simulink library "inp_BCKP"  (R2021b)
settings: Solver=VariableStepAuto  StartTime=0.0  StopTime=10.0  RelTol=1e-3
undefined symbols (not defined in the file): C_TASK_5MS_S, FALSE, KINP_AcoreReadyToSlp_flg_ovrdflg, KINP_AcoreReadyToSlp_flg_ovrdval, KINP_AllowMovThd_OTA_enum_ovrdflg, KINP_AllowMovThd_OTA_enum_ovrdval, KINP_APSAngleTarget_Deg_ovrdflg, KINP_APSAngleTarget_Deg_ovrdval, KINP_APSDecReq_mps2_ovrdflg, KINP_APSDecReq_mps2_ovrdval, KINP_APSDecReqA_flg_ovrdflg, KINP_APSDecReqA_flg_ovrdval, KINP_APSDFLL_cm_ovrdflg, KINP_APSDFLL_cm_ovrdval, KINP_APSDFLR_cm_ovrdflg, KINP_APSDFLR_cm_ovrdval, KINP_APSDRLL_cm_ovrdflg, KINP_APSDRLL_cm_ovrdval, KINP_APSDRLR_cm_ovrdflg, KINP_APSDRLR_cm_ovrdval, KINP_APSExitCondition_enum_ovrdflg, KINP_APSExitCondition_enum_ovrdval, KINP_APSHWVer_enum_ovrdflg, KINP_APSHWVer_enum_ovrdval, KINP_APSProgressPCT_pct_ovrdflg, KINP_APSProgressPCT_pct_ovrdval, KINP_APSPwrReq_enum_ovrdflg, KINP_APSPwrReq_enum_ovrdval, KINP_APSReq_enum_ovrdflg, KINP_APSReq_enum_ovrdval, KINP_APSRQDisplay_enum_ovrdflg, KINP_APSRQDisplay_enum_ovrdval, KINP_APSRqEPASCtrl_flg_ovrdflg, KINP_APSRqEPASCtrl_flg_ovrdval, KINP_APSShiftPosnReq_enum_ovrdval, KINP_APSShiftPosnReq_enum_ovrflg, KINP_APSSpeedCMD_kph_ovrdval, KINP_APSSpeedCMD_kph_ovrflg, KINP_APSStaSystem_enum_ovrdflg, KINP_APSStaSystem_enum_ovrdval, KINP_APSSWVer_enum_ovrdflg, KINP_APSSWVer_enum_ovrdval, KINP_APSVMCReqA_flg_ovrdval, KINP_APSVMCReqA_flg_ovrflg, KINP_APSVRqEPASCtrl_flg_ovrdflg, KINP_APSVRqEPASCtrl_flg_ovrdval, KINP_AuxBattVolmV_mV_ovrdflg, KINP_AuxBattVolmV_mV_ovrdval, KINP_BTConnectSta_enum_ovrdflg, KINP_BTConnectSta_enum_ovrdval, KINP_CAASSta_enum_ovrdflg, KINP_CAASSta_enum_ovrdval, KINP_CAASVMCReqA_flg_ovrdval, KINP_CAASVMCReqA_flg_ovrflg, KINP_CAN1BusOff_flg_ovrdflg, KINP_CAN1BusOff_flg_ovrdval, KINP_CAN2BusOff_flg_ovrdflg, KINP_CAN2BusOff_flg_ovrdval, KINP_CAN3BusOff_flg_ovrdflg, KINP_CAN3BusOff_flg_ovrdval ... (+158)
libraries: FVT_lib x144, hcu_lib x1
(part 6 of 8)

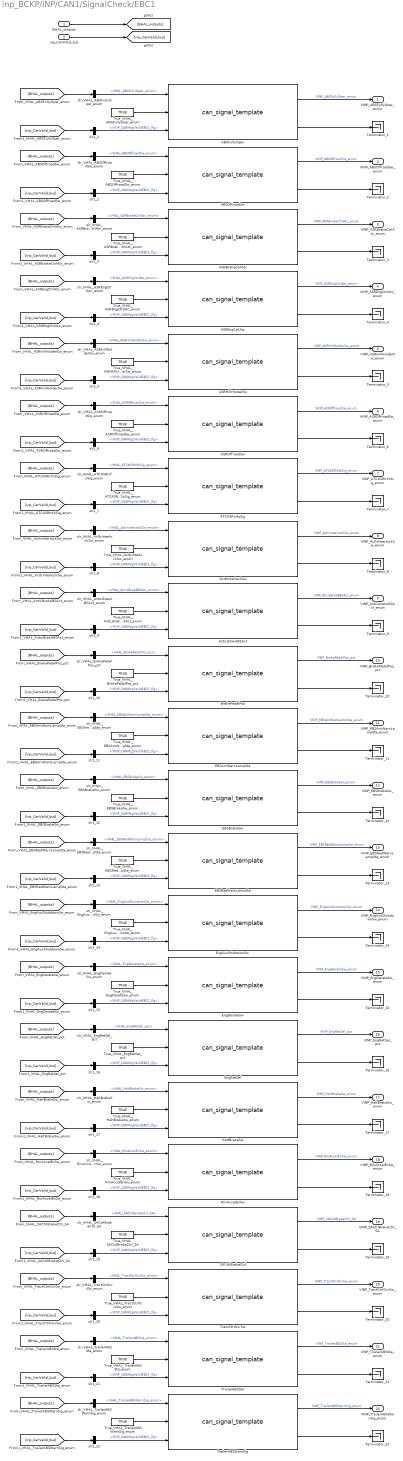
== system inp_BCKP/INP/CAN1/SignalCheck/EBC1 ==
  BHAL_outputs : Inport
  inp_CanValid_bus : Inport  Port=2
  ABSFullyOper : FVT_lib/inp/can_signal_template  SystemSampleTime=-1  VariantActivationTime=update diagram  Latency=0  AutoFrameSizeCalculation=off
      link override defval: Value=KINP_ABSFullyOper_enum_defval
      link override ovrdflg: Value=KINP_ABSFullyOper_enum_ovrdflg
      link override ovrdval: Value=KINP_ABSFullyOper_enum_ovrdval
  ABSOffroadSw : FVT_lib/inp/can_signal_template  SystemSampleTime=-1  VariantActivationTime=update diagram  Latency=0  AutoFrameSizeCalculation=off
      link override defval: Value=KINP_ABSOffroadSw_enum_defval
      link override ovrdflg: Value=KINP_ABSOffroadSw_enum_ovrdflg
      link override ovrdval: Value=KINP_ABSOffroadSw_enum_ovrdval
  ASRBrakeCtrlAtc : FVT_lib/inp/can_signal_template  SystemSampleTime=-1  VariantActivationTime=update diagram  Latency=0  AutoFrameSizeCalculation=off
      link override defval: Value=KINP_ASRBrakeCtrlAtc_enum_defval
      link override ovrdflg: Value=KINP_ASRBrakeCtrlAtc_enum_ovrdflg
      link override ovrdval: Value=KINP_ASRBrakeCtrlAtc_enum_ovrdval
  ASREngCtrlAtc : FVT_lib/inp/can_signal_template  SystemSampleTime=-1  VariantActivationTime=update diagram  Latency=0  AutoFrameSizeCalculation=off
      link override defval: Value=KINP_ASREngCtrlAtc_enum_defval
      link override ovrdflg: Value=KINP_ASREngCtrlAtc_enum_ovrdflg
      link override ovrdval: Value=KINP_ASREngCtrlAtc_enum_ovrdval
  ASRHillHolderSw : FVT_lib/inp/can_signal_template  SystemSampleTime=-1  VariantActivationTime=update diagram  Latency=0  AutoFrameSizeCalculation=off
      link override defval: Value=KINP_ASRHillHolderSw_enum_defval
      link override ovrdflg: Value=KINP_ASRHillHolderSw_enum_ovrdflg
      link override ovrdval: Value=KINP_ASRHillHolderSw_enum_ovrdval
  ASROffroadSw : FVT_lib/inp/can_signal_template  SystemSampleTime=-1  VariantActivationTime=update diagram  Latency=0  AutoFrameSizeCalculation=off
      link override defval: Value=KINP_ASROffroadSw_enum_defval
      link override ovrdflg: Value=KINP_ASROffroadSw_enum_ovrdflg
      link override ovrdval: Value=KINP_ASROffroadSw_enum_ovrdval
  ATCASRInfoSig : FVT_lib/inp/can_signal_template  SystemSampleTime=-1  VariantActivationTime=update diagram  Latency=0  AutoFrameSizeCalculation=off
      link override defval: Value=KINP_ATCASRInfoSig_enum_defval
      link override ovrdflg: Value=KINP_ATCASRInfoSig_enum_ovrdflg
      link override ovrdval: Value=KINP_ATCASRInfoSig_enum_ovrdval
  AcltrInterlockSw : FVT_lib/inp/can_signal_template  SystemSampleTime=-1  VariantActivationTime=update diagram  Latency=0  AutoFrameSizeCalculation=off
      link override defval: Value=KINP_AcltrInterlockSw_enum_defval
      link override ovrdflg: Value=KINP_AcltrInterlockSw_enum_ovrdflg
      link override ovrdval: Value=KINP_AcltrInterlockSw_enum_ovrdval
  AntiLBrakABSAct : FVT_lib/inp/can_signal_template  SystemSampleTime=-1  VariantActivationTime=update diagram  Latency=0  AutoFrameSizeCalculation=off
      link override defval: Value=KINP_AntiLBrakABSAct_enum_defval
      link override ovrdflg: Value=KINP_AntiLBrakABSAct_enum_ovrdflg
      link override ovrdval: Value=KINP_AntiLBrakABSAct_enum_ovrdval
  BrakePedalPos : FVT_lib/inp/can_signal_template  SystemSampleTime=-1  VariantActivationTime=update diagram  Latency=0  AutoFrameSizeCalculation=off
      link override defval: Value=KINP_BrakePedalPos_pct_defval
      link override ovrdflg: Value=KINP_BrakePedalPos_pct_ovrdflg
      link override ovrdval: Value=KINP_BrakePedalPos_pct_ovrdval
  EBSAmWarnLampSta : FVT_lib/inp/can_signal_template  SystemSampleTime=-1  VariantActivationTime=update diagram  Latency=0  AutoFrameSizeCalculation=off
      link override defval: Value=KINP_EBSAmWarnLampSta_enum_defval
      link override ovrdflg: Value=KINP_EBSAmWarnLampSta_enum_ovrdflg
      link override ovrdval: Value=KINP_EBSAmWarnLampSta_enum_ovrdval
  EBSBrakeSw : FVT_lib/inp/can_signal_template  SystemSampleTime=-1  VariantActivationTime=update diagram  Latency=0  AutoFrameSizeCalculation=off
      link override defval: Value=KINP_EBSBrakeSw_enum_defval
      link override ovrdflg: Value=KINP_EBSBrakeSw_enum_ovrdflg
      link override ovrdval: Value=KINP_EBSBrakeSw_enum_ovrdval
  EBSRedWarnLampSta : FVT_lib/inp/can_signal_template  SystemSampleTime=-1  VariantActivationTime=update diagram  Latency=0  AutoFrameSizeCalculation=off
      link override defval: Value=KINP_EBSRedWarnLampSta_enum_defval
      link override ovrdflg: Value=KINP_EBSRedWarnLampSta_enum_ovrdflg
      link override ovrdval: Value=KINP_EBSRedWarnLampSta_enum_ovrdval
  EngAuxShutdownSw : FVT_lib/inp/can_signal_template  SystemSampleTime=-1  VariantActivationTime=update diagram  Latency=0  AutoFrameSizeCalculation=off
      link override defval: Value=KINP_EngAuxShutdownSw_enum_defval
      link override ovrdflg: Value=KINP_EngAuxShutdownSw_enum_ovrdflg
      link override ovrdval: Value=KINP_EngAuxShutdownSw_enum_ovrdval
  EngDerateSw : FVT_lib/inp/can_signal_template  SystemSampleTime=-1  VariantActivationTime=update diagram  Latency=0  AutoFrameSizeCalculation=off
      link override defval: Value=KINP_EngDerateSw_enum_defval
      link override ovrdflg: Value=KINP_EngDerateSw_enum_ovrdflg
      link override ovrdval: Value=KINP_EngDerateSw_enum_ovrdval
  EngRetSel : FVT_lib/inp/can_signal_template  SystemSampleTime=-1  VariantActivationTime=update diagram  Latency=0  AutoFrameSizeCalculation=off
      link override defval: Value=KINP_EngRetSel_pct_defval
      link override ovrdflg: Value=KINP_EngRetSel_pct_ovrdflg
      link override ovrdval: Value=KINP_EngRetSel_pct_ovrdval
  HaltBrakeSw : FVT_lib/inp/can_signal_template  SystemSampleTime=-1  VariantActivationTime=update diagram  Latency=0  AutoFrameSizeCalculation=off
      link override defval: Value=KINP_HaltBrakeSw_enum_defval
      link override ovrdflg: Value=KINP_HaltBrakeSw_enum_ovrdflg
      link override ovrdval: Value=KINP_HaltBrakeSw_enum_ovrdval
  RmAccelEnSw : FVT_lib/inp/can_signal_template  SystemSampleTime=-1  VariantActivationTime=update diagram  Latency=0  AutoFrameSizeCalculation=off
      link override defval: Value=KINP_RmAccelEnSw_enum_defval
      link override ovrdflg: Value=KINP_RmAccelEnSw_enum_ovrdflg
      link override ovrdval: Value=KINP_RmAccelEnSw_enum_ovrdval
  SACtrlBrakeCtrl : FVT_lib/inp/can_signal_template  SystemSampleTime=-1  VariantActivationTime=update diagram  Latency=0  AutoFrameSizeCalculation=off
      link override defval: Value=KINP_SACtrlBrakeCtrl_SA_defval
      link override ovrdflg: Value=KINP_SACtrlBrakeCtrl_SA_ovrdflg
      link override ovrdval: Value=KINP_SACtrlBrakeCtrl_SA_ovrdval
  Terminator_{1..22} (22 alike) : Terminator
  TractCtrlOvrSw : FVT_lib/inp/can_signal_template  SystemSampleTime=-1  VariantActivationTime=update diagram  Latency=0  AutoFrameSizeCalculation=off
      link override defval: Value=KINP_TractCtrlOvrSw_enum_defval
      link override ovrdflg: Value=KINP_TractCtrlOvrSw_enum_ovrdflg
      link override ovrdval: Value=KINP_TractCtrlOvrSw_enum_ovrdval
  TrailerABSSta : FVT_lib/inp/can_signal_template  SystemSampleTime=-1  VariantActivationTime=update diagram  Latency=0  AutoFrameSizeCalculation=off
      link override defval: Value=KINP_TrailerABSSta_enum_defval
      link override ovrdflg: Value=KINP_TrailerABSSta_enum_ovrdflg
      link override ovrdval: Value=KINP_TrailerABSSta_enum_ovrdval
  TrailerABSWarnSig : FVT_lib/inp/can_signal_template  SystemSampleTime=-1  VariantActivationTime=update diagram  Latency=0  AutoFrameSizeCalculation=off
      link override defval: Value=KINP_TrailerABSWarnSig_enum_defval
      link override ovrdflg: Value=KINP_TrailerABSWarnSig_enum_ovrdflg
      link override ovrdval: Value=KINP_TrailerABSWarnSig_enum_ovrdval
  True_VHAL_ABSFullyOper_enum : Constant  Value=TRUE  OutDataTypeStr=boolean
  True_VHAL_ABSOffroadSw_enum : Constant  Value=TRUE  OutDataTypeStr=boolean
  True_VHAL_ASRBrakeCtrlAtc_enum : Constant  Value=TRUE  OutDataTypeStr=boolean
  True_VHAL_ASREngCtrlAtc_enum : Constant  Value=TRUE  OutDataTypeStr=boolean
  True_VHAL_ASRHillHolderSw_enum : Constant  Value=TRUE  OutDataTypeStr=boolean
  True_VHAL_ASROffroadSw_enum : Constant  Value=TRUE  OutDataTypeStr=boolean
  True_VHAL_ATCASRInfoSig_enum : Constant  Value=TRUE  OutDataTypeStr=boolean
  True_VHAL_AcltrInterlockSw_enum : Constant  Value=TRUE  OutDataTypeStr=boolean
  True_VHAL_AntiLBrakABSAct_enum : Constant  Value=TRUE  OutDataTypeStr=boolean
  True_VHAL_BrakePedalPos_pct : Constant  Value=TRUE  OutDataTypeStr=boolean
  True_VHAL_EBSAmWarnLampSta_enum : Constant  Value=TRUE  OutDataTypeStr=boolean
  True_VHAL_EBSBrakeSw_enum : Constant  Value=TRUE  OutDataTypeStr=boolean
  True_VHAL_EBSRedWarnLampSta_enum : Constant  Value=TRUE  OutDataTypeStr=boolean
  True_VHAL_EngAuxShutdownSw_enum : Constant  Value=TRUE  OutDataTypeStr=boolean
  True_VHAL_EngDerateSw_enum : Constant  Value=TRUE  OutDataTypeStr=boolean
  True_VHAL_EngRetSel_pct : Constant  Value=TRUE  OutDataTypeStr=boolean
  True_VHAL_HaltBrakeSw_enum : Constant  Value=TRUE  OutDataTypeStr=boolean
  True_VHAL_RmAccelEnSw_enum : Constant  Value=TRUE  OutDataTypeStr=boolean
  True_VHAL_SACtrlBrakeCtrl_SA : Constant  Value=TRUE  OutDataTypeStr=boolean
  True_VHAL_TractCtrlOvrSw_enum : Constant  Value=TRUE  OutDataTypeStr=boolean
  True_VHAL_TrailerABSSta_enum : Constant  Value=TRUE  OutDataTypeStr=boolean
  True_VHAL_TrailerABSWarnSig_enum : Constant  Value=TRUE  OutDataTypeStr=boolean
  slr1_{1..22} (22 alike) : BusSelector  OutputSignals=VINP_CANMsgValidEBC1_flg
  slr_VHAL_ABSFullyOper_enum : BusSelector  OutputSignals=VHAL_ABSFullyOper_enum
  slr_VHAL_ABSOffroadSw_enum : BusSelector  OutputSignals=VHAL_ABSOffroadSw_enum
  slr_VHAL_ASRBrakeCtrlAtc_enum : BusSelector  OutputSignals=VHAL_ASRBrakeCtrlAtc_enum
  slr_VHAL_ASREngCtrlAtc_enum : BusSelector  OutputSignals=VHAL_ASREngCtrlAtc_enum
  slr_VHAL_ASRHillHolderSw_enum : BusSelector  OutputSignals=VHAL_ASRHillHolderSw_enum
  slr_VHAL_ASROffroadSw_enum : BusSelector  OutputSignals=VHAL_ASROffroadSw_enum
  slr_VHAL_ATCASRInfoSig_enum : BusSelector  OutputSignals=VHAL_ATCASRInfoSig_enum
  slr_VHAL_AcltrInterlockSw_enum : BusSelector  OutputSignals=VHAL_AcltrInterlockSw_enum
  slr_VHAL_AntiLBrakABSAct_enum : BusSelector  OutputSignals=VHAL_AntiLBrakABSAct_enum
  slr_VHAL_BrakePedalPos_pct : BusSelector  OutputSignals=VHAL_BrakePedalPos_pct
  slr_VHAL_EBSAmWarnLampSta_enum : BusSelector  OutputSignals=VHAL_EBSAmWarnLampSta_enum
  slr_VHAL_EBSBrakeSw_enum : BusSelector  OutputSignals=VHAL_EBSBrakeSw_enum
  slr_VHAL_EBSRedWarnLampSta_enum : BusSelector  OutputSignals=VHAL_EBSRedWarnLampSta_enum
  slr_VHAL_EngAuxShutdownSw_enum : BusSelector  OutputSignals=VHAL_EngAuxShutdownSw_enum
  slr_VHAL_EngDerateSw_enum : BusSelector  OutputSignals=VHAL_EngDerateSw_enum
  slr_VHAL_EngRetSel_pct : BusSelector  OutputSignals=VHAL_EngRetSel_pct
  slr_VHAL_HaltBrakeSw_enum : BusSelector  OutputSignals=VHAL_HaltBrakeSw_enum
  slr_VHAL_RmAccelEnSw_enum : BusSelector  OutputSignals=VHAL_RmAccelEnSw_enum
  slr_VHAL_SACtrlBrakeCtrl_SA : BusSelector  OutputSignals=VHAL_SACtrlBrakeCtrl_SA
  slr_VHAL_TractCtrlOvrSw_enum : BusSelector  OutputSignals=VHAL_TractCtrlOvrSw_enum
  slr_VHAL_TrailerABSSta_enum : BusSelector  OutputSignals=VHAL_TrailerABSSta_enum
  slr_VHAL_TrailerABSWarnSig_enum : BusSelector  OutputSignals=VHAL_TrailerABSWarnSig_enum
  VINP_ABSFullyOper_enum : Outport
  VINP_ABSOffroadSw_enum : Outport  Port=2
  VINP_ASRBrakeCtrlAtc_enum : Outport  Port=3
  VINP_ASREngCtrlAtc_enum : Outport  Port=4
  VINP_ASRHillHolderSw_enum : Outport  Port=5
  VINP_ASROffroadSw_enum : Outport  Port=6
  VINP_ATCASRInfoSig_enum : Outport  Port=7
  VINP_AcltrInterlockSw_enum : Outport  Port=8
  VINP_AntiLBrakABSAct_enum : Outport  Port=9
  VINP_BrakePedalPos_pct : Outport  Port=10
  VINP_EBSAmWarnLampSta_enum : Outport  Port=11
  VINP_EBSBrakeSw_enum : Outport  Port=12
  VINP_EBSRedWarnLampSta_enum : Outport  Port=13
  VINP_EngAuxShutdownSw_enum : Outport  Port=14
  VINP_EngDerateSw_enum : Outport  Port=15
  VINP_EngRetSel_pct : Outport  Port=16
  VINP_HaltBrakeSw_enum : Outport  Port=17
  VINP_RmAccelEnSw_enum : Outport  Port=18
  VINP_SACtrlBrakeCtrl_SA : Outport  Port=19
  VINP_TractCtrlOvrSw_enum : Outport  Port=20
  VINP_TrailerABSSta_enum : Outport  Port=21
  VINP_TrailerABSWarnSig_enum : Outport  Port=22
  wires:
  BHAL_outputs/1 -> [BHAL_outputs]
  inp_CanValid_bus/1 -> [inp_CanValid_bus]
  [BHAL_outputs] -> slr_VHAL_ABSFullyOper_enum/1
  slr_VHAL_ABSFullyOper_enum/1 -> ABSFullyOper/1  "<VHAL_ABSFullyOper_enum>"
  True_VHAL_ABSFullyOper_enum/1 -> ABSFullyOper/2
  [inp_CanValid_bus] -> slr1_1/1
  slr1_1/1 -> ABSFullyOper/3  "<VINP_CANMsgValidEBC1_flg>"
  ABSFullyOper/1 -> VINP_ABSFullyOper_enum/1  "VINP_ABSFullyOper_enum"
  ABSFullyOper/2 -> Terminator_1/1
  [BHAL_outputs] -> slr_VHAL_ABSOffroadSw_enum/1
  slr_VHAL_ABSOffroadSw_enum/1 -> ABSOffroadSw/1  "<VHAL_ABSOffroadSw_enum>"
  True_VHAL_ABSOffroadSw_enum/1 -> ABSOffroadSw/2
  [inp_CanValid_bus] -> slr1_2/1
  slr1_2/1 -> ABSOffroadSw/3  "<VINP_CANMsgValidEBC1_flg>"
  ABSOffroadSw/1 -> VINP_ABSOffroadSw_enum/1  "VINP_ABSOffroadSw_enum"
  ABSOffroadSw/2 -> Terminator_2/1
  [BHAL_outputs] -> slr_VHAL_ASRBrakeCtrlAtc_enum/1
  slr_VHAL_ASRBrakeCtrlAtc_enum/1 -> ASRBrakeCtrlAtc/1  "<VHAL_ASRBrakeCtrlAtc_enum>"
  True_VHAL_ASRBrakeCtrlAtc_enum/1 -> ASRBrakeCtrlAtc/2
  [inp_CanValid_bus] -> slr1_3/1
  slr1_3/1 -> ASRBrakeCtrlAtc/3  "<VINP_CANMsgValidEBC1_flg>"
  ASRBrakeCtrlAtc/1 -> VINP_ASRBrakeCtrlAtc_enum/1  "VINP_ASRBrakeCtrlAtc_enum"
  ASRBrakeCtrlAtc/2 -> Terminator_3/1
  [BHAL_outputs] -> slr_VHAL_ASREngCtrlAtc_enum/1
  slr_VHAL_ASREngCtrlAtc_enum/1 -> ASREngCtrlAtc/1  "<VHAL_ASREngCtrlAtc_enum>"
  True_VHAL_ASREngCtrlAtc_enum/1 -> ASREngCtrlAtc/2
  [inp_CanValid_bus] -> slr1_4/1
  slr1_4/1 -> ASREngCtrlAtc/3  "<VINP_CANMsgValidEBC1_flg>"
  ASREngCtrlAtc/1 -> VINP_ASREngCtrlAtc_enum/1  "VINP_ASREngCtrlAtc_enum"
  ASREngCtrlAtc/2 -> Terminator_4/1
  [BHAL_outputs] -> slr_VHAL_ASRHillHolderSw_enum/1
  slr_VHAL_ASRHillHolderSw_enum/1 -> ASRHillHolderSw/1  "<VHAL_ASRHillHolderSw_enum>"
  True_VHAL_ASRHillHolderSw_enum/1 -> ASRHillHolderSw/2
  [inp_CanValid_bus] -> slr1_5/1
  slr1_5/1 -> ASRHillHolderSw/3  "<VINP_CANMsgValidEBC1_flg>"
  ASRHillHolderSw/1 -> VINP_ASRHillHolderSw_enum/1  "VINP_ASRHillHolderSw_enum"
  ASRHillHolderSw/2 -> Terminator_5/1
  [BHAL_outputs] -> slr_VHAL_ASROffroadSw_enum/1
  slr_VHAL_ASROffroadSw_enum/1 -> ASROffroadSw/1  "<VHAL_ASROffroadSw_enum>"
  True_VHAL_ASROffroadSw_enum/1 -> ASROffroadSw/2
  [inp_CanValid_bus] -> slr1_6/1
  slr1_6/1 -> ASROffroadSw/3  "<VINP_CANMsgValidEBC1_flg>"
  ASROffroadSw/1 -> VINP_ASROffroadSw_enum/1  "VINP_ASROffroadSw_enum"
  ASROffroadSw/2 -> Terminator_6/1
  [BHAL_outputs] -> slr_VHAL_ATCASRInfoSig_enum/1
  slr_VHAL_ATCASRInfoSig_enum/1 -> ATCASRInfoSig/1  "<VHAL_ATCASRInfoSig_enum>"
  True_VHAL_ATCASRInfoSig_enum/1 -> ATCASRInfoSig/2
  [inp_CanValid_bus] -> slr1_7/1
  slr1_7/1 -> ATCASRInfoSig/3  "<VINP_CANMsgValidEBC1_flg>"
  ATCASRInfoSig/1 -> VINP_ATCASRInfoSig_enum/1  "VINP_ATCASRInfoSig_enum"
  ATCASRInfoSig/2 -> Terminator_7/1
  [BHAL_outputs] -> slr_VHAL_AcltrInterlockSw_enum/1
  slr_VHAL_AcltrInterlockSw_enum/1 -> AcltrInterlockSw/1  "<VHAL_AcltrInterlockSw_enum>"
  True_VHAL_AcltrInterlockSw_enum/1 -> AcltrInterlockSw/2
  [inp_CanValid_bus] -> slr1_8/1
  slr1_8/1 -> AcltrInterlockSw/3  "<VINP_CANMsgValidEBC1_flg>"
  AcltrInterlockSw/1 -> VINP_AcltrInterlockSw_enum/1  "VINP_AcltrInterlockSw_enum"
  AcltrInterlockSw/2 -> Terminator_8/1
  [BHAL_outputs] -> slr_VHAL_AntiLBrakABSAct_enum/1
  slr_VHAL_AntiLBrakABSAct_enum/1 -> AntiLBrakABSAct/1  "<VHAL_AntiLBrakABSAct_enum>"
  True_VHAL_AntiLBrakABSAct_enum/1 -> AntiLBrakABSAct/2
  [inp_CanValid_bus] -> slr1_9/1
  slr1_9/1 -> AntiLBrakABSAct/3  "<VINP_CANMsgValidEBC1_flg>"
  AntiLBrakABSAct/1 -> VINP_AntiLBrakABSAct_enum/1  "VINP_AntiLBrakABSAct_enum"
  AntiLBrakABSAct/2 -> Terminator_9/1
  [BHAL_outputs] -> slr_VHAL_BrakePedalPos_pct/1
  slr_VHAL_BrakePedalPos_pct/1 -> BrakePedalPos/1  "<VHAL_BrakePedalPos_pct>"
  True_VHAL_BrakePedalPos_pct/1 -> BrakePedalPos/2
  [inp_CanValid_bus] -> slr1_10/1
  slr1_10/1 -> BrakePedalPos/3  "<VINP_CANMsgValidEBC1_flg>"
  BrakePedalPos/1 -> VINP_BrakePedalPos_pct/1  "VINP_BrakePedalPos_pct"
  BrakePedalPos/2 -> Terminator_10/1
  [BHAL_outputs] -> slr_VHAL_EBSAmWarnLampSta_enum/1
  slr_VHAL_EBSAmWarnLampSta_enum/1 -> EBSAmWarnLampSta/1  "<VHAL_EBSAmWarnLampSta_enum>"
  True_VHAL_EBSAmWarnLampSta_enum/1 -> EBSAmWarnLampSta/2
  [inp_CanValid_bus] -> slr1_11/1
  slr1_11/1 -> EBSAmWarnLampSta/3  "<VINP_CANMsgValidEBC1_flg>"
  EBSAmWarnLampSta/1 -> VINP_EBSAmWarnLampSta_enum/1  "VINP_EBSAmWarnLampSta_enum"
  EBSAmWarnLampSta/2 -> Terminator_11/1
  [BHAL_outputs] -> slr_VHAL_EBSBrakeSw_enum/1
  slr_VHAL_EBSBrakeSw_enum/1 -> EBSBrakeSw/1  "<VHAL_EBSBrakeSw_enum>"
  True_VHAL_EBSBrakeSw_enum/1 -> EBSBrakeSw/2
  [inp_CanValid_bus] -> slr1_12/1
  slr1_12/1 -> EBSBrakeSw/3  "<VINP_CANMsgValidEBC1_flg>"
  EBSBrakeSw/1 -> VINP_EBSBrakeSw_enum/1  "VINP_EBSBrakeSw_enum"
  EBSBrakeSw/2 -> Terminator_12/1
  [BHAL_outputs] -> slr_VHAL_EBSRedWarnLampSta_enum/1
  slr_VHAL_EBSRedWarnLampSta_enum/1 -> EBSRedWarnLampSta/1  "<VHAL_EBSRedWarnLampSta_enum>"
  True_VHAL_EBSRedWarnLampSta_enum/1 -> EBSRedWarnLampSta/2
  [inp_CanValid_bus] -> slr1_13/1
  slr1_13/1 -> EBSRedWarnLampSta/3  "<VINP_CANMsgValidEBC1_flg>"
  EBSRedWarnLampSta/1 -> VINP_EBSRedWarnLampSta_enum/1  "VINP_EBSRedWarnLampSta_enum"
  EBSRedWarnLampSta/2 -> Terminator_13/1
  [BHAL_outputs] -> slr_VHAL_EngAuxShutdownSw_enum/1
  slr_VHAL_EngAuxShutdownSw_enum/1 -> EngAuxShutdownSw/1  "<VHAL_EngAuxShutdownSw_enum>"
  True_VHAL_EngAuxShutdownSw_enum/1 -> EngAuxShutdownSw/2
  [inp_CanValid_bus] -> slr1_14/1
  slr1_14/1 -> EngAuxShutdownSw/3  "<VINP_CANMsgValidEBC1_flg>"
  EngAuxShutdownSw/1 -> VINP_EngAuxShutdownSw_enum/1  "VINP_EngAuxShutdownSw_enum"
  EngAuxShutdownSw/2 -> Terminator_14/1
  [BHAL_outputs] -> slr_VHAL_EngDerateSw_enum/1
  slr_VHAL_EngDerateSw_enum/1 -> EngDerateSw/1  "<VHAL_EngDerateSw_enum>"
  True_VHAL_EngDerateSw_enum/1 -> EngDerateSw/2
  [inp_CanValid_bus] -> slr1_15/1
  slr1_15/1 -> EngDerateSw/3  "<VINP_CANMsgValidEBC1_flg>"
  EngDerateSw/1 -> VINP_EngDerateSw_enum/1  "VINP_EngDerateSw_enum"
  EngDerateSw/2 -> Terminator_15/1
  [BHAL_outputs] -> slr_VHAL_EngRetSel_pct/1
  slr_VHAL_EngRetSel_pct/1 -> EngRetSel/1  "<VHAL_EngRetSel_pct>"
  True_VHAL_EngRetSel_pct/1 -> EngRetSel/2
  [inp_CanValid_bus] -> slr1_16/1
  slr1_16/1 -> EngRetSel/3  "<VINP_CANMsgValidEBC1_flg>"
  EngRetSel/1 -> VINP_EngRetSel_pct/1  "VINP_EngRetSel_pct"
  EngRetSel/2 -> Terminator_16/1
  [BHAL_outputs] -> slr_VHAL_HaltBrakeSw_enum/1
  slr_VHAL_HaltBrakeSw_enum/1 -> HaltBrakeSw/1  "<VHAL_HaltBrakeSw_enum>"
  True_VHAL_HaltBrakeSw_enum/1 -> HaltBrakeSw/2
  [inp_CanValid_bus] -> slr1_17/1
  slr1_17/1 -> HaltBrakeSw/3  "<VINP_CANMsgValidEBC1_flg>"
  HaltBrakeSw/1 -> VINP_HaltBrakeSw_enum/1  "VINP_HaltBrakeSw_enum"
  HaltBrakeSw/2 -> Terminator_17/1
  [BHAL_outputs] -> slr_VHAL_RmAccelEnSw_enum/1
  slr_VHAL_RmAccelEnSw_enum/1 -> RmAccelEnSw/1  "<VHAL_RmAccelEnSw_enum>"
  True_VHAL_RmAccelEnSw_enum/1 -> RmAccelEnSw/2
  [inp_CanValid_bus] -> slr1_18/1
  slr1_18/1 -> RmAccelEnSw/3  "<VINP_CANMsgValidEBC1_flg>"
  RmAccelEnSw/1 -> VINP_RmAccelEnSw_enum/1  "VINP_RmAccelEnSw_enum"
  RmAccelEnSw/2 -> Terminator_18/1
  [BHAL_outputs] -> slr_VHAL_SACtrlBrakeCtrl_SA/1
  slr_VHAL_SACtrlBrakeCtrl_SA/1 -> SACtrlBrakeCtrl/1  "<VHAL_SACtrlBrakeCtrl_SA>"
  True_VHAL_SACtrlBrakeCtrl_SA/1 -> SACtrlBrakeCtrl/2
  [inp_CanValid_bus] -> slr1_19/1
  slr1_19/1 -> SACtrlBrakeCtrl/3  "<VINP_CANMsgValidEBC1_flg>"
  SACtrlBrakeCtrl/1 -> VINP_SACtrlBrakeCtrl_SA/1  "VINP_SACtrlBrakeCtrl_SA"
  SACtrlBrakeCtrl/2 -> Terminator_19/1
  [BHAL_outputs] -> slr_VHAL_TractCtrlOvrSw_enum/1
  slr_VHAL_TractCtrlOvrSw_enum/1 -> TractCtrlOvrSw/1  "<VHAL_TractCtrlOvrSw_enum>"
  True_VHAL_TractCtrlOvrSw_enum/1 -> TractCtrlOvrSw/2
  [inp_CanValid_bus] -> slr1_20/1
  slr1_20/1 -> TractCtrlOvrSw/3  "<VINP_CANMsgValidEBC1_flg>"
  TractCtrlOvrSw/1 -> VINP_TractCtrlOvrSw_enum/1  "VINP_TractCtrlOvrSw_enum"
  TractCtrlOvrSw/2 -> Terminator_20/1
  [BHAL_outputs] -> slr_VHAL_TrailerABSSta_enum/1
  slr_VHAL_TrailerABSSta_enum/1 -> TrailerABSSta/1  "<VHAL_TrailerABSSta_enum>"
  True_VHAL_TrailerABSSta_enum/1 -> TrailerABSSta/2
  [inp_CanValid_bus] -> slr1_21/1
  slr1_21/1 -> TrailerABSSta/3  "<VINP_CANMsgValidEBC1_flg>"
  TrailerABSSta/1 -> VINP_TrailerABSSta_enum/1  "VINP_TrailerABSSta_enum"
  TrailerABSSta/2 -> Terminator_21/1
  [BHAL_outputs] -> slr_VHAL_TrailerABSWarnSig_enum/1
  slr_VHAL_TrailerABSWarnSig_enum/1 -> TrailerABSWarnSig/1  "<VHAL_TrailerABSWarnSig_enum>"
  True_VHAL_TrailerABSWarnSig_enum/1 -> TrailerABSWarnSig/2
  [inp_CanValid_bus] -> slr1_22/1
  slr1_22/1 -> TrailerABSWarnSig/3  "<VINP_CANMsgValidEBC1_flg>"
  TrailerABSWarnSig/1 -> VINP_TrailerABSWarnSig_enum/1  "VINP_TrailerABSWarnSig_enum"
  TrailerABSWarnSig/2 -> Terminator_22/1

== system inp_BCKP/INP/CAN1/SignalCheck/EBC2 ==
  BHAL_outputs : Inport
  inp_CanValid_bus : Inport  Port=2
  FASpeed : FVT_lib/inp/can_signal_template  SystemSampleTime=-1  VariantActivationTime=update diagram  Latency=0  AutoFrameSizeCalculation=off
      link override defval: Value=KINP_FASpeed_kph_defval
      link override ovrdflg: Value=KINP_FASpeed_kph_ovrdflg
      link override ovrdval: Value=KINP_FASpeed_kph_ovrdval
  RelaSpdFALWheel : FVT_lib/inp/can_signal_template  SystemSampleTime=-1  VariantActivationTime=update diagram  Latency=0  AutoFrameSizeCalculation=off
      link override defval: Value=KINP_RelaSpdFALWheel_kph_defval
      link override ovrdflg: Value=KINP_RelaSpdFALWheel_kph_ovrdflg
      link override ovrdval: Value=KINP_RelaSpdFALWheel_kph_ovrdval
  RelaSpdFARWheel : FVT_lib/inp/can_signal_template  SystemSampleTime=-1  VariantActivationTime=update diagram  Latency=0  AutoFrameSizeCalculation=off
      link override defval: Value=KINP_RelaSpdFARWheel_kph_defval
      link override ovrdflg: Value=KINP_RelaSpdFARWheel_kph_ovrdflg
      link override ovrdval: Value=KINP_RelaSpdFARWheel_kph_ovrdval
  Terminator_1 : Terminator
  Terminator_2 : Terminator
  Terminator_3 : Terminator
  True_VHAL_FASpeed_kph : Constant  Value=TRUE  OutDataTypeStr=boolean
  True_VHAL_RelaSpdFALWheel_kph : Constant  Value=TRUE  OutDataTypeStr=boolean
  True_VHAL_RelaSpdFARWheel_kph : Constant  Value=TRUE  OutDataTypeStr=boolean
  slr1_1 : BusSelector  OutputSignals=VINP_CANMsgValidEBC2_flg
  slr1_2 : BusSelector  OutputSignals=VINP_CANMsgValidEBC2_flg
  slr1_3 : BusSelector  OutputSignals=VINP_CANMsgValidEBC2_flg
  slr_VHAL_FASpeed_kph : BusSelector  OutputSignals=VHAL_FASpeed_kph
  slr_VHAL_RelaSpdFALWheel_kph : BusSelector  OutputSignals=VHAL_RelaSpdFALWheel_kph
  slr_VHAL_RelaSpdFARWheel_kph : BusSelector  OutputSignals=VHAL_RelaSpdFARWheel_kph
  VINP_FASpeed_kph : Outport
  VINP_RelaSpdFALWheel_kph : Outport  Port=2
  VINP_RelaSpdFARWheel_kph : Outport  Port=3
  wires:
  BHAL_outputs/1 -> [BHAL_outputs]
  inp_CanValid_bus/1 -> [inp_CanValid_bus]
  [BHAL_outputs] -> slr_VHAL_FASpeed_kph/1
  slr_VHAL_FASpeed_kph/1 -> FASpeed/1  "<VHAL_FASpeed_kph>"
  True_VHAL_FASpeed_kph/1 -> FASpeed/2
  [inp_CanValid_bus] -> slr1_1/1
  slr1_1/1 -> FASpeed/3  "<VINP_CANMsgValidEBC2_flg>"
  FASpeed/1 -> VINP_FASpeed_kph/1  "VINP_FASpeed_kph"
  FASpeed/2 -> Terminator_1/1
  [BHAL_outputs] -> slr_VHAL_RelaSpdFALWheel_kph/1
  slr_VHAL_RelaSpdFALWheel_kph/1 -> RelaSpdFALWheel/1  "<VHAL_RelaSpdFALWheel_kph>"
  True_VHAL_RelaSpdFALWheel_kph/1 -> RelaSpdFALWheel/2
  [inp_CanValid_bus] -> slr1_2/1
  slr1_2/1 -> RelaSpdFALWheel/3  "<VINP_CANMsgValidEBC2_flg>"
  RelaSpdFALWheel/1 -> VINP_RelaSpdFALWheel_kph/1  "VINP_RelaSpdFALWheel_kph"
  RelaSpdFALWheel/2 -> Terminator_2/1
  [BHAL_outputs] -> slr_VHAL_RelaSpdFARWheel_kph/1
  slr_VHAL_RelaSpdFARWheel_kph/1 -> RelaSpdFARWheel/1  "<VHAL_RelaSpdFARWheel_kph>"
  True_VHAL_RelaSpdFARWheel_kph/1 -> RelaSpdFARWheel/2
  [inp_CanValid_bus] -> slr1_3/1
  slr1_3/1 -> RelaSpdFARWheel/3  "<VINP_CANMsgValidEBC2_flg>"
  RelaSpdFARWheel/1 -> VINP_RelaSpdFARWheel_kph/1  "VINP_RelaSpdFARWheel_kph"
  RelaSpdFARWheel/2 -> Terminator_3/1

== system inp_BCKP/INP/CAN1/SignalCheck/EBC5 ==
  BHAL_outputs : Inport
  inp_CanValid_bus : Inport  Port=2
  BrkTempeWarn : FVT_lib/inp/can_signal_template  SystemSampleTime=-1  VariantActivationTime=update diagram  Latency=0  AutoFrameSizeCalculation=off
      link override defval: Value=KINP_BrkTempeWarn_enum_defval
      link override ovrdflg: Value=KINP_BrkTempeWarn_enum_ovrdflg
      link override ovrdval: Value=KINP_BrkTempeWarn_enum_ovrdval
  FndBrkUse : FVT_lib/inp/can_signal_template  SystemSampleTime=-1  VariantActivationTime=update diagram  Latency=0  AutoFrameSizeCalculation=off
      link override defval: Value=KINP_FndBrkUse_enum_defval
      link override ovrdflg: Value=KINP_FndBrkUse_enum_ovrdflg
      link override ovrdval: Value=KINP_FndBrkUse_enum_ovrdval
  HaltBrkMode : FVT_lib/inp/can_signal_template  SystemSampleTime=-1  VariantActivationTime=update diagram  Latency=0  AutoFrameSizeCalculation=off
      link override defval: Value=KINP_HaltBrkMode_enum_defval
      link override ovrdflg: Value=KINP_HaltBrkMode_enum_ovrdflg
      link override ovrdval: Value=KINP_HaltBrkMode_enum_ovrdval
  HillHolderMode : FVT_lib/inp/can_signal_template  SystemSampleTime=-1  VariantActivationTime=update diagram  Latency=0  AutoFrameSizeCalculation=off
      link override defval: Value=KINP_HillHolderMode_enum_defval
      link override ovrdflg: Value=KINP_HillHolderMode_enum_ovrdflg
      link override ovrdval: Value=KINP_HillHolderMode_enum_ovrdval
  ParkBrkActuFAct : FVT_lib/inp/can_signal_template  SystemSampleTime=-1  VariantActivationTime=update diagram  Latency=0  AutoFrameSizeCalculation=off
      link override defval: Value=KINP_ParkBrkActuFAct_enum_defval
      link override ovrdflg: Value=KINP_ParkBrkActuFAct_enum_ovrdflg
      link override ovrdval: Value=KINP_ParkBrkActuFAct_enum_ovrdval
  Terminator_{1..8} (8 alike) : Terminator
  True_VHAL_BrkTempeWarn_enum : Constant  Value=TRUE  OutDataTypeStr=boolean
  True_VHAL_FndBrkUse_enum : Constant  Value=TRUE  OutDataTypeStr=boolean
  True_VHAL_HaltBrkMode_enum : Constant  Value=TRUE  OutDataTypeStr=boolean
  True_VHAL_HillHolderMode_enum : Constant  Value=TRUE  OutDataTypeStr=boolean
  True_VHAL_ParkBrkActuFAct_enum : Constant  Value=TRUE  OutDataTypeStr=boolean
  True_VHAL_XBRAcltnLimit_mps2 : Constant  Value=TRUE  OutDataTypeStr=boolean
  True_VHAL_XBRActtrlMode_enum : Constant  Value=TRUE  OutDataTypeStr=boolean
  True_VHAL_XBRSysSta_enum : Constant  Value=TRUE  OutDataTypeStr=boolean
  XBRAcltnLimit : FVT_lib/inp/can_signal_template  SystemSampleTime=-1  VariantActivationTime=update diagram  Latency=0  AutoFrameSizeCalculation=off
      link override defval: Value=KINP_XBRAcltnLimit_mps2_defval
      link override ovrdflg: Value=KINP_XBRAcltnLimit_mps2_ovrdflg
      link override ovrdval: Value=KINP_XBRAcltnLimit_mps2_ovrdval
  XBRActtrlMode : FVT_lib/inp/can_signal_template  SystemSampleTime=-1  VariantActivationTime=update diagram  Latency=0  AutoFrameSizeCalculation=off
      link override defval: Value=KINP_XBRActtrlMode_enum_defval
      link override ovrdflg: Value=KINP_XBRActtrlMode_enum_ovrdflg
      link override ovrdval: Value=KINP_XBRActtrlMode_enum_ovrdval
  XBRSysSta : FVT_lib/inp/can_signal_template  SystemSampleTime=-1  VariantActivationTime=update diagram  Latency=0  AutoFrameSizeCalculation=off
      link override defval: Value=KINP_XBRSysSta_enum_defval
      link override ovrdflg: Value=KINP_XBRSysSta_enum_ovrdflg
      link override ovrdval: Value=KINP_XBRSysSta_enum_ovrdval
  slr1_{1..8} (8 alike) : BusSelector  OutputSignals=VINP_CANMsgValidEBC5_flg
  slr_VHAL_BrkTempeWarn_enum : BusSelector  OutputSignals=VHAL_BrkTempeWarn_enum
  slr_VHAL_FndBrkUse_enum : BusSelector  OutputSignals=VHAL_FndBrkUse_enum
  slr_VHAL_HaltBrkMode_enum : BusSelector  OutputSignals=VHAL_HaltBrkMode_enum
  slr_VHAL_HillHolderMode_enum : BusSelector  OutputSignals=VHAL_HillHolderMode_enum
  slr_VHAL_ParkBrkActuFAct_enum : BusSelector  OutputSignals=VHAL_ParkBrkActuFAct_enum
  slr_VHAL_XBRAcltnLimit_mps2 : BusSelector  OutputSignals=VHAL_XBRAcltnLimit_mps2
  slr_VHAL_XBRActtrlMode_enum : BusSelector  OutputSignals=VHAL_XBRActtrlMode_enum
  slr_VHAL_XBRSysSta_enum : BusSelector  OutputSignals=VHAL_XBRSysSta_enum
  VINP_BrkTempeWarn_enum : Outport
  VINP_FndBrkUse_enum : Outport  Port=2
  VINP_HaltBrkMode_enum : Outport  Port=3
  VINP_HillHolderMode_enum : Outport  Port=4
  VINP_ParkBrkActuFAct_enum : Outport  Port=5
  VINP_XBRAcltnLimit_mps2 : Outport  Port=6
  VINP_XBRActtrlMode_enum : Outport  Port=7
  VINP_XBRSysSta_enum : Outport  Port=8
  wires:
  BHAL_outputs/1 -> [BHAL_outputs]
  inp_CanValid_bus/1 -> [inp_CanValid_bus]
  [BHAL_outputs] -> slr_VHAL_BrkTempeWarn_enum/1
  slr_VHAL_BrkTempeWarn_enum/1 -> BrkTempeWarn/1  "<VHAL_BrkTempeWarn_enum>"
  True_VHAL_BrkTempeWarn_enum/1 -> BrkTempeWarn/2
  [inp_CanValid_bus] -> slr1_1/1
  slr1_1/1 -> BrkTempeWarn/3  "<VINP_CANMsgValidEBC5_flg>"
  BrkTempeWarn/1 -> VINP_BrkTempeWarn_enum/1  "VINP_BrkTempeWarn_enum"
  BrkTempeWarn/2 -> Terminator_1/1
  [BHAL_outputs] -> slr_VHAL_FndBrkUse_enum/1
  slr_VHAL_FndBrkUse_enum/1 -> FndBrkUse/1  "<VHAL_FndBrkUse_enum>"
  True_VHAL_FndBrkUse_enum/1 -> FndBrkUse/2
  [inp_CanValid_bus] -> slr1_2/1
  slr1_2/1 -> FndBrkUse/3  "<VINP_CANMsgValidEBC5_flg>"
  FndBrkUse/1 -> VINP_FndBrkUse_enum/1  "VINP_FndBrkUse_enum"
  FndBrkUse/2 -> Terminator_2/1
  [BHAL_outputs] -> slr_VHAL_HaltBrkMode_enum/1
  slr_VHAL_HaltBrkMode_enum/1 -> HaltBrkMode/1  "<VHAL_HaltBrkMode_enum>"
  True_VHAL_HaltBrkMode_enum/1 -> HaltBrkMode/2
  [inp_CanValid_bus] -> slr1_3/1
  slr1_3/1 -> HaltBrkMode/3  "<VINP_CANMsgValidEBC5_flg>"
  HaltBrkMode/1 -> VINP_HaltBrkMode_enum/1  "VINP_HaltBrkMode_enum"
  HaltBrkMode/2 -> Terminator_3/1
  [BHAL_outputs] -> slr_VHAL_HillHolderMode_enum/1
  slr_VHAL_HillHolderMode_enum/1 -> HillHolderMode/1  "<VHAL_HillHolderMode_enum>"
  True_VHAL_HillHolderMode_enum/1 -> HillHolderMode/2
  [inp_CanValid_bus] -> slr1_4/1
  slr1_4/1 -> HillHolderMode/3  "<VINP_CANMsgValidEBC5_flg>"
  HillHolderMode/1 -> VINP_HillHolderMode_enum/1  "VINP_HillHolderMode_enum"
  HillHolderMode/2 -> Terminator_4/1
  [BHAL_outputs] -> slr_VHAL_ParkBrkActuFAct_enum/1
  slr_VHAL_ParkBrkActuFAct_enum/1 -> ParkBrkActuFAct/1  "<VHAL_ParkBrkActuFAct_enum>"
  True_VHAL_ParkBrkActuFAct_enum/1 -> ParkBrkActuFAct/2
  [inp_CanValid_bus] -> slr1_5/1
  slr1_5/1 -> ParkBrkActuFAct/3  "<VINP_CANMsgValidEBC5_flg>"
  ParkBrkActuFAct/1 -> VINP_ParkBrkActuFAct_enum/1  "VINP_ParkBrkActuFAct_enum"
  ParkBrkActuFAct/2 -> Terminator_5/1
  [BHAL_outputs] -> slr_VHAL_XBRAcltnLimit_mps2/1
  slr_VHAL_XBRAcltnLimit_mps2/1 -> XBRAcltnLimit/1  "<VHAL_XBRAcltnLimit_mps2>"
  True_VHAL_XBRAcltnLimit_mps2/1 -> XBRAcltnLimit/2
  [inp_CanValid_bus] -> slr1_6/1
  slr1_6/1 -> XBRAcltnLimit/3  "<VINP_CANMsgValidEBC5_flg>"
  XBRAcltnLimit/1 -> VINP_XBRAcltnLimit_mps2/1  "VINP_XBRAcltnLimit_mps2"
  XBRAcltnLimit/2 -> Terminator_6/1
  [BHAL_outputs] -> slr_VHAL_XBRActtrlMode_enum/1
  slr_VHAL_XBRActtrlMode_enum/1 -> XBRActtrlMode/1  "<VHAL_XBRActtrlMode_enum>"
  True_VHAL_XBRActtrlMode_enum/1 -> XBRActtrlMode/2
  [inp_CanValid_bus] -> slr1_7/1
  slr1_7/1 -> XBRActtrlMode/3  "<VINP_CANMsgValidEBC5_flg>"
  XBRActtrlMode/1 -> VINP_XBRActtrlMode_enum/1  "VINP_XBRActtrlMode_enum"
  XBRActtrlMode/2 -> Terminator_7/1
  [BHAL_outputs] -> slr_VHAL_XBRSysSta_enum/1
  slr_VHAL_XBRSysSta_enum/1 -> XBRSysSta/1  "<VHAL_XBRSysSta_enum>"
  True_VHAL_XBRSysSta_enum/1 -> XBRSysSta/2
  [inp_CanValid_bus] -> slr1_8/1
  slr1_8/1 -> XBRSysSta/3  "<VINP_CANMsgValidEBC5_flg>"
  XBRSysSta/1 -> VINP_XBRSysSta_enum/1  "VINP_XBRSysSta_enum"
  XBRSysSta/2 -> Terminator_8/1

== system inp_BCKP/INP/CAN1/SignalCheck/ECAS_DM1 ==
  BHAL_outputs : Inport
  inp_CanValid_bus : Inport  Port=2
  ECASAWarmLampSta : FVT_lib/inp/can_signal_template  SystemSampleTime=-1  VariantActivationTime=update diagram  Latency=0  AutoFrameSizeCalculation=off
      link override defval: Value=KINP_ECASAWarmLampSta_enum_defval
      link override ovrdflg: Value=KINP_ECASAWarmLampSta_enum_ovrdflg
      link override ovrdval: Value=KINP_ECASAWarmLampSta_enum_ovrdval
  Terminator_1 : Terminator
  True_VHAL_ECASAWarmLampSta_enum : Constant  Value=TRUE  OutDataTypeStr=boolean
  slr1_1 : BusSelector  OutputSignals=VINP_CANMsgValidECASDM1_flg
  slr_VHAL_ECASAWarmLampSta_enum : BusSelector  OutputSignals=VHAL_ECASAWarmLampSta_enum
  VINP_ECASAWarmLampSta_enum : Outport
  wires:
  BHAL_outputs/1 -> [BHAL_outputs]
  inp_CanValid_bus/1 -> [inp_CanValid_bus]
  [BHAL_outputs] -> slr_VHAL_ECASAWarmLampSta_enum/1
  slr_VHAL_ECASAWarmLampSta_enum/1 -> ECASAWarmLampSta/1  "<VHAL_ECASAWarmLampSta_enum>"
  True_VHAL_ECASAWarmLampSta_enum/1 -> ECASAWarmLampSta/2
  [inp_CanValid_bus] -> slr1_1/1
  slr1_1/1 -> ECASAWarmLampSta/3  "<VINP_CANMsgValidECASDM1_flg>"
  ECASAWarmLampSta/1 -> VINP_ECASAWarmLampSta_enum/1  "VINP_ECASAWarmLampSta_enum"
  ECASAWarmLampSta/2 -> Terminator_1/1

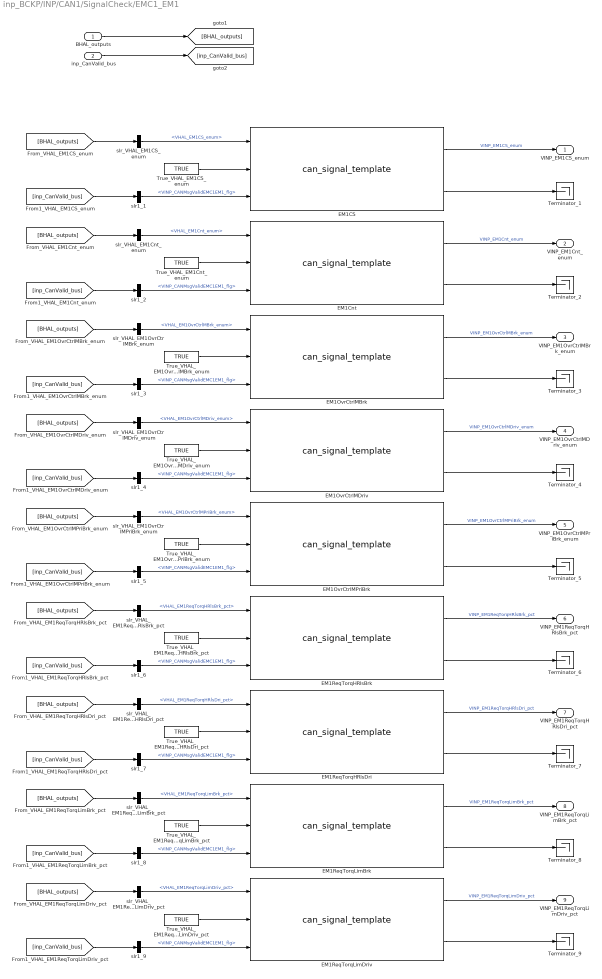
== system inp_BCKP/INP/CAN1/SignalCheck/EMC1_EM1 ==
  BHAL_outputs : Inport
  inp_CanValid_bus : Inport  Port=2
  EM1CS : FVT_lib/inp/can_signal_template  SystemSampleTime=-1  VariantActivationTime=update diagram  Latency=0  AutoFrameSizeCalculation=off
      link override defval: Value=KINP_EM1CS_enum_defval
      link override ovrdflg: Value=KINP_EM1CS_enum_ovrdflg
      link override ovrdval: Value=KINP_EM1CS_enum_ovrdval
  EM1Cnt : FVT_lib/inp/can_signal_template  SystemSampleTime=-1  VariantActivationTime=update diagram  Latency=0  AutoFrameSizeCalculation=off
      link override defval: Value=KINP_EM1Cnt_enum_defval
      link override ovrdflg: Value=KINP_EM1Cnt_enum_ovrdflg
      link override ovrdval: Value=KINP_EM1Cnt_enum_ovrdval
  EM1OvrCtrlMBrk : FVT_lib/inp/can_signal_template  SystemSampleTime=-1  VariantActivationTime=update diagram  Latency=0  AutoFrameSizeCalculation=off
      link override defval: Value=KINP_EM1OvrCtrlMBrk_enum_defval
      link override ovrdflg: Value=KINP_EM1OvrCtrlMBrk_enum_ovrdflg
      link override ovrdval: Value=KINP_EM1OvrCtrlMBrk_enum_ovrdval
  EM1OvrCtrlMDriv : FVT_lib/inp/can_signal_template  SystemSampleTime=-1  VariantActivationTime=update diagram  Latency=0  AutoFrameSizeCalculation=off
      link override defval: Value=KINP_EM1OvrCtrlMDriv_enum_defval
      link override ovrdflg: Value=KINP_EM1OvrCtrlMDriv_enum_ovrdflg
      link override ovrdval: Value=KINP_EM1OvrCtrlMDriv_enum_ovrdval
  EM1OvrCtrlMPriBrk : FVT_lib/inp/can_signal_template  SystemSampleTime=-1  VariantActivationTime=update diagram  Latency=0  AutoFrameSizeCalculation=off
      link override defval: Value=KINP_EM1OvrCtrlMPriBrk_enum_defval
      link override ovrdflg: Value=KINP_EM1OvrCtrlMPriBrk_enum_ovrdflg
      link override ovrdval: Value=KINP_EM1OvrCtrlMPriBrk_enum_ovrdval
  EM1ReqTorqHRlsBrk : FVT_lib/inp/can_signal_template  SystemSampleTime=-1  VariantActivationTime=update diagram  Latency=0  AutoFrameSizeCalculation=off
      link override defval: Value=KINP_EM1ReqTorqHRlsBrk_pct_defval
      link override ovrdflg: Value=KINP_EM1ReqTorqHRlsBrk_pct_ovrdflg
      link override ovrdval: Value=KINP_EM1ReqTorqHRlsBrk_pct_ovrdval
  EM1ReqTorqHRlsDri : FVT_lib/inp/can_signal_template  SystemSampleTime=-1  VariantActivationTime=update diagram  Latency=0  AutoFrameSizeCalculation=off
      link override defval: Value=KINP_EM1ReqTorqHRlsDri_pct_defval
      link override ovrdflg: Value=KINP_EM1ReqTorqHRlsDri_pct_ovrdflg
      link override ovrdval: Value=KINP_EM1ReqTorqHRlsDri_pct_ovrdval
  EM1ReqTorqLimBrk : FVT_lib/inp/can_signal_template  SystemSampleTime=-1  VariantActivationTime=update diagram  Latency=0  AutoFrameSizeCalculation=off
      link override defval: Value=KINP_EM1ReqTorqLimBrk_pct_defval
      link override ovrdflg: Value=KINP_EM1ReqTorqLimBrk_pct_ovrdflg
      link override ovrdval: Value=KINP_EM1ReqTorqLimBrk_pct_ovrdval
  EM1ReqTorqLimDriv : FVT_lib/inp/can_signal_template  SystemSampleTime=-1  VariantActivationTime=update diagram  Latency=0  AutoFrameSizeCalculation=off
      link override defval: Value=KINP_EM1ReqTorqLimDriv_pct_defval
      link override ovrdflg: Value=KINP_EM1ReqTorqLimDriv_pct_ovrdflg
      link override ovrdval: Value=KINP_EM1ReqTorqLimDriv_pct_ovrdval
  Terminator_{1..9} (9 alike) : Terminator
  True_VHAL_EM1CS_enum : Constant  Value=TRUE  OutDataTypeStr=boolean
  True_VHAL_EM1Cnt_enum : Constant  Value=TRUE  OutDataTypeStr=boolean
  True_VHAL_EM1OvrCtrlMBrk_enum : Constant  Value=TRUE  OutDataTypeStr=boolean
  True_VHAL_EM1OvrCtrlMDriv_enum : Constant  Value=TRUE  OutDataTypeStr=boolean
  True_VHAL_EM1OvrCtrlMPriBrk_enum : Constant  Value=TRUE  OutDataTypeStr=boolean
  True_VHAL_EM1ReqTorqHRlsBrk_pct : Constant  Value=TRUE  OutDataTypeStr=boolean
  True_VHAL_EM1ReqTorqHRlsDri_pct : Constant  Value=TRUE  OutDataTypeStr=boolean
  True_VHAL_EM1ReqTorqLimBrk_pct : Constant  Value=TRUE  OutDataTypeStr=boolean
  True_VHAL_EM1ReqTorqLimDriv_pct : Constant  Value=TRUE  OutDataTypeStr=boolean
  slr1_{1..9} (9 alike) : BusSelector  OutputSignals=VINP_CANMsgValidEMC1EM1_flg
  slr_VHAL_EM1CS_enum : BusSelector  OutputSignals=VHAL_EM1CS_enum
  slr_VHAL_EM1Cnt_enum : BusSelector  OutputSignals=VHAL_EM1Cnt_enum
  slr_VHAL_EM1OvrCtrlMBrk_enum : BusSelector  OutputSignals=VHAL_EM1OvrCtrlMBrk_enum
  slr_VHAL_EM1OvrCtrlMDriv_enum : BusSelector  OutputSignals=VHAL_EM1OvrCtrlMDriv_enum
  slr_VHAL_EM1OvrCtrlMPriBrk_enum : BusSelector  OutputSignals=VHAL_EM1OvrCtrlMPriBrk_enum
  slr_VHAL_EM1ReqTorqHRlsBrk_pct : BusSelector  OutputSignals=VHAL_EM1ReqTorqHRlsBrk_pct
  slr_VHAL_EM1ReqTorqHRlsDri_pct : BusSelector  OutputSignals=VHAL_EM1ReqTorqHRlsDri_pct
  slr_VHAL_EM1ReqTorqLimBrk_pct : BusSelector  OutputSignals=VHAL_EM1ReqTorqLimBrk_pct
  slr_VHAL_EM1ReqTorqLimDriv_pct : BusSelector  OutputSignals=VHAL_EM1ReqTorqLimDriv_pct
  VINP_EM1CS_enum : Outport
  VINP_EM1Cnt_enum : Outport  Port=2
  VINP_EM1OvrCtrlMBrk_enum : Outport  Port=3
  VINP_EM1OvrCtrlMDriv_enum : Outport  Port=4
  VINP_EM1OvrCtrlMPriBrk_enum : Outport  Port=5
  VINP_EM1ReqTorqHRlsBrk_pct : Outport  Port=6
  VINP_EM1ReqTorqHRlsDri_pct : Outport  Port=7
  VINP_EM1ReqTorqLimBrk_pct : Outport  Port=8
  VINP_EM1ReqTorqLimDriv_pct : Outport  Port=9
  wires:
  BHAL_outputs/1 -> [BHAL_outputs]
  inp_CanValid_bus/1 -> [inp_CanValid_bus]
  [BHAL_outputs] -> slr_VHAL_EM1CS_enum/1
  slr_VHAL_EM1CS_enum/1 -> EM1CS/1  "<VHAL_EM1CS_enum>"
  True_VHAL_EM1CS_enum/1 -> EM1CS/2
  [inp_CanValid_bus] -> slr1_1/1
  slr1_1/1 -> EM1CS/3  "<VINP_CANMsgValidEMC1EM1_flg>"
  EM1CS/1 -> VINP_EM1CS_enum/1  "VINP_EM1CS_enum"
  EM1CS/2 -> Terminator_1/1
  [BHAL_outputs] -> slr_VHAL_EM1Cnt_enum/1
  slr_VHAL_EM1Cnt_enum/1 -> EM1Cnt/1  "<VHAL_EM1Cnt_enum>"
  True_VHAL_EM1Cnt_enum/1 -> EM1Cnt/2
  [inp_CanValid_bus] -> slr1_2/1
  slr1_2/1 -> EM1Cnt/3  "<VINP_CANMsgValidEMC1EM1_flg>"
  EM1Cnt/1 -> VINP_EM1Cnt_enum/1  "VINP_EM1Cnt_enum"
  EM1Cnt/2 -> Terminator_2/1
  [BHAL_outputs] -> slr_VHAL_EM1OvrCtrlMBrk_enum/1
  slr_VHAL_EM1OvrCtrlMBrk_enum/1 -> EM1OvrCtrlMBrk/1  "<VHAL_EM1OvrCtrlMBrk_enum>"
  True_VHAL_EM1OvrCtrlMBrk_enum/1 -> EM1OvrCtrlMBrk/2
  [inp_CanValid_bus] -> slr1_3/1
  slr1_3/1 -> EM1OvrCtrlMBrk/3  "<VINP_CANMsgValidEMC1EM1_flg>"
  EM1OvrCtrlMBrk/1 -> VINP_EM1OvrCtrlMBrk_enum/1  "VINP_EM1OvrCtrlMBrk_enum"
  EM1OvrCtrlMBrk/2 -> Terminator_3/1
  [BHAL_outputs] -> slr_VHAL_EM1OvrCtrlMDriv_enum/1
  slr_VHAL_EM1OvrCtrlMDriv_enum/1 -> EM1OvrCtrlMDriv/1  "<VHAL_EM1OvrCtrlMDriv_enum>"
  True_VHAL_EM1OvrCtrlMDriv_enum/1 -> EM1OvrCtrlMDriv/2
  [inp_CanValid_bus] -> slr1_4/1
  slr1_4/1 -> EM1OvrCtrlMDriv/3  "<VINP_CANMsgValidEMC1EM1_flg>"
  EM1OvrCtrlMDriv/1 -> VINP_EM1OvrCtrlMDriv_enum/1  "VINP_EM1OvrCtrlMDriv_enum"
  EM1OvrCtrlMDriv/2 -> Terminator_4/1
  [BHAL_outputs] -> slr_VHAL_EM1OvrCtrlMPriBrk_enum/1
  slr_VHAL_EM1OvrCtrlMPriBrk_enum/1 -> EM1OvrCtrlMPriBrk/1  "<VHAL_EM1OvrCtrlMPriBrk_enum>"
  True_VHAL_EM1OvrCtrlMPriBrk_enum/1 -> EM1OvrCtrlMPriBrk/2
  [inp_CanValid_bus] -> slr1_5/1
  slr1_5/1 -> EM1OvrCtrlMPriBrk/3  "<VINP_CANMsgValidEMC1EM1_flg>"
  EM1OvrCtrlMPriBrk/1 -> VINP_EM1OvrCtrlMPriBrk_enum/1  "VINP_EM1OvrCtrlMPriBrk_enum"
  EM1OvrCtrlMPriBrk/2 -> Terminator_5/1
  [BHAL_outputs] -> slr_VHAL_EM1ReqTorqHRlsBrk_pct/1
  slr_VHAL_EM1ReqTorqHRlsBrk_pct/1 -> EM1ReqTorqHRlsBrk/1  "<VHAL_EM1ReqTorqHRlsBrk_pct>"
  True_VHAL_EM1ReqTorqHRlsBrk_pct/1 -> EM1ReqTorqHRlsBrk/2
  [inp_CanValid_bus] -> slr1_6/1
  slr1_6/1 -> EM1ReqTorqHRlsBrk/3  "<VINP_CANMsgValidEMC1EM1_flg>"
  EM1ReqTorqHRlsBrk/1 -> VINP_EM1ReqTorqHRlsBrk_pct/1  "VINP_EM1ReqTorqHRlsBrk_pct"
  EM1ReqTorqHRlsBrk/2 -> Terminator_6/1
  [BHAL_outputs] -> slr_VHAL_EM1ReqTorqHRlsDri_pct/1
  slr_VHAL_EM1ReqTorqHRlsDri_pct/1 -> EM1ReqTorqHRlsDri/1  "<VHAL_EM1ReqTorqHRlsDri_pct>"
  True_VHAL_EM1ReqTorqHRlsDri_pct/1 -> EM1ReqTorqHRlsDri/2
  [inp_CanValid_bus] -> slr1_7/1
  slr1_7/1 -> EM1ReqTorqHRlsDri/3  "<VINP_CANMsgValidEMC1EM1_flg>"
  EM1ReqTorqHRlsDri/1 -> VINP_EM1ReqTorqHRlsDri_pct/1  "VINP_EM1ReqTorqHRlsDri_pct"
  EM1ReqTorqHRlsDri/2 -> Terminator_7/1
  [BHAL_outputs] -> slr_VHAL_EM1ReqTorqLimBrk_pct/1
  slr_VHAL_EM1ReqTorqLimBrk_pct/1 -> EM1ReqTorqLimBrk/1  "<VHAL_EM1ReqTorqLimBrk_pct>"
  True_VHAL_EM1ReqTorqLimBrk_pct/1 -> EM1ReqTorqLimBrk/2
  [inp_CanValid_bus] -> slr1_8/1
  slr1_8/1 -> EM1ReqTorqLimBrk/3  "<VINP_CANMsgValidEMC1EM1_flg>"
  EM1ReqTorqLimBrk/1 -> VINP_EM1ReqTorqLimBrk_pct/1  "VINP_EM1ReqTorqLimBrk_pct"
  EM1ReqTorqLimBrk/2 -> Terminator_8/1
  [BHAL_outputs] -> slr_VHAL_EM1ReqTorqLimDriv_pct/1
  slr_VHAL_EM1ReqTorqLimDriv_pct/1 -> EM1ReqTorqLimDriv/1  "<VHAL_EM1ReqTorqLimDriv_pct>"
  True_VHAL_EM1ReqTorqLimDriv_pct/1 -> EM1ReqTorqLimDriv/2
  [inp_CanValid_bus] -> slr1_9/1
  slr1_9/1 -> EM1ReqTorqLimDriv/3  "<VINP_CANMsgValidEMC1EM1_flg>"
  EM1ReqTorqLimDriv/1 -> VINP_EM1ReqTorqLimDriv_pct/1  "VINP_EM1ReqTorqLimDriv_pct"
  EM1ReqTorqLimDriv/2 -> Terminator_9/1

== system inp_BCKP/INP/CAN1/SignalCheck/HRW ==
  BHAL_outputs : Inport
  inp_CanValid_bus : Inport  Port=2
  Terminator_1 : Terminator
  True_VHAL_WhlSpeedFL_kph : Constant  Value=TRUE  OutDataTypeStr=boolean
  WhlSpeedFL : FVT_lib/inp/can_signal_template  SystemSampleTime=-1  VariantActivationTime=update diagram  Latency=0  AutoFrameSizeCalculation=off
      link override defval: Value=KINP_WhlSpeedFL_kph_defval
      link override ovrdflg: Value=KINP_WhlSpeedFL_kph_ovrdflg
      link override ovrdval: Value=KINP_WhlSpeedFL_kph_ovrdval
  slr1_1 : BusSelector  OutputSignals=VINP_CANMsgValidHRW_flg
  slr_VHAL_WhlSpeedFL_kph : BusSelector  OutputSignals=VHAL_WhlSpeedFL_kph
  VINP_WhlSpeedFL_kph : Outport
  wires:
  BHAL_outputs/1 -> [BHAL_outputs]
  inp_CanValid_bus/1 -> [inp_CanValid_bus]
  [BHAL_outputs] -> slr_VHAL_WhlSpeedFL_kph/1
  slr_VHAL_WhlSpeedFL_kph/1 -> WhlSpeedFL/1  "<VHAL_WhlSpeedFL_kph>"
  True_VHAL_WhlSpeedFL_kph/1 -> WhlSpeedFL/2
  [inp_CanValid_bus] -> slr1_1/1
  slr1_1/1 -> WhlSpeedFL/3  "<VINP_CANMsgValidHRW_flg>"
  WhlSpeedFL/1 -> VINP_WhlSpeedFL_kph/1  "VINP_WhlSpeedFL_kph"
  WhlSpeedFL/2 -> Terminator_1/1

== system inp_BCKP/INP/CAN1/SignalCheck/TC1 ==
  BHAL_outputs : Inport
  inp_CanValid_bus : Inport  Port=2
  DrivDirF : FVT_lib/inp/can_signal_template  SystemSampleTime=-1  VariantActivationTime=update diagram  Latency=0  AutoFrameSizeCalculation=off
      link override defval: Value=KINP_DrivDirF_enum_defval
      link override ovrdflg: Value=KINP_DrivDirF_enum_ovrdflg
      link override ovrdval: Value=KINP_DrivDirF_enum_ovrdval
  Terminator_1 : Terminator
  Terminator_2 : Terminator
  TransReqGear : FVT_lib/inp/can_signal_template  SystemSampleTime=-1  VariantActivationTime=update diagram  Latency=0  AutoFrameSizeCalculation=off
      link override defval: Value=KINP_TransReqGear_enum_defval
      link override ovrdflg: Value=KINP_TransReqGear_enum_ovrdflg
      link override ovrdval: Value=KINP_TransReqGear_enum_ovrdval
  True_VHAL_DrivDirF_enum : Constant  Value=TRUE  OutDataTypeStr=boolean
  True_VHAL_TransReqGear_enum : Constant  Value=TRUE  OutDataTypeStr=boolean
  slr1_1 : BusSelector  OutputSignals=VINP_CANMsgValidTC1_flg
  slr1_2 : BusSelector  OutputSignals=VINP_CANMsgValidTC1_flg
  slr_VHAL_DrivDirF_enum : BusSelector  OutputSignals=VHAL_DrivDirF_enum
  slr_VHAL_TransReqGear_enum : BusSelector  OutputSignals=VHAL_TransReqGear_enum
  VINP_DrivDirF_enum : Outport
  VINP_TransReqGear_enum : Outport  Port=2
  wires:
  BHAL_outputs/1 -> [BHAL_outputs]
  inp_CanValid_bus/1 -> [inp_CanValid_bus]
  [BHAL_outputs] -> slr_VHAL_DrivDirF_enum/1
  slr_VHAL_DrivDirF_enum/1 -> DrivDirF/1  "<VHAL_DrivDirF_enum>"
  True_VHAL_DrivDirF_enum/1 -> DrivDirF/2
  [inp_CanValid_bus] -> slr1_1/1
  slr1_1/1 -> DrivDirF/3  "<VINP_CANMsgValidTC1_flg>"
  DrivDirF/1 -> VINP_DrivDirF_enum/1  "VINP_DrivDirF_enum"
  DrivDirF/2 -> Terminator_1/1
  [BHAL_outputs] -> slr_VHAL_TransReqGear_enum/1
  slr_VHAL_TransReqGear_enum/1 -> TransReqGear/1  "<VHAL_TransReqGear_enum>"
  True_VHAL_TransReqGear_enum/1 -> TransReqGear/2
  [inp_CanValid_bus] -> slr1_2/1
  slr1_2/1 -> TransReqGear/3  "<VINP_CANMsgValidTC1_flg>"
  TransReqGear/1 -> VINP_TransReqGear_enum/1  "VINP_TransReqGear_enum"
  TransReqGear/2 -> Terminator_2/1

== system inp_BCKP/INP/CAN2/SignalCheck/IVI_C100_0 ==
  BHAL_outputs : Inport
  inp_CanValid_bus : Inport  Port=2
  IVIACFanSpdReqCmd : FVT_lib/inp/can_signal_template  SystemSampleTime=-1  VariantActivationTime=update diagram  Latency=0  AutoFrameSizeCalculation=off
      link override defval: Value=KINP_IVIACFanSpdReqCmd_enum_defval
      link override ovrdflg: Value=KINP_IVIACFanSpdReqCmd_enum_ovrdflg
      link override ovrdval: Value=KINP_IVIACFanSpdReqCmd_enum_ovrdval
  Terminator_1 : Terminator
  True_VHAL_IVIACFanSpdReqCmd_enum : Constant  Value=TRUE  OutDataTypeStr=boolean
  slr1_1 : BusSelector  OutputSignals=VINP_CANMsgValidIVIC1000_flg
  slr_VHAL_IVIACFanSpdReqCmd_enum : BusSelector  OutputSignals=VHAL_IVIACFanSpdReqCmd_enum
  VINP_IVIACFanSpdReqCmd_enum : Outport
  wires:
  BHAL_outputs/1 -> [BHAL_outputs]
  inp_CanValid_bus/1 -> [inp_CanValid_bus]
  [BHAL_outputs] -> slr_VHAL_IVIACFanSpdReqCmd_enum/1
  slr_VHAL_IVIACFanSpdReqCmd_enum/1 -> IVIACFanSpdReqCmd/1  "<VHAL_IVIACFanSpdReqCmd_enum>"
  True_VHAL_IVIACFanSpdReqCmd_enum/1 -> IVIACFanSpdReqCmd/2
  [inp_CanValid_bus] -> slr1_1/1
  slr1_1/1 -> IVIACFanSpdReqCmd/3  "<VINP_CANMsgValidIVIC1000_flg>"
  IVIACFanSpdReqCmd/1 -> VINP_IVIACFanSpdReqCmd_enum/1  "VINP_IVIACFanSpdReqCmd_enum"
  IVIACFanSpdReqCmd/2 -> Terminator_1/1
